simulink model "poly_festk2"  (Simulink 7.8)
settings: Solver=VariableStepDiscrete  StartTime=0.0  StopTime=100  RelTol=1e-3
undefined symbols (not defined in the file or in its folder): get
libraries: dspsigops x2, dspmlti4 x2, dspstat3 x1, dspsnks4 x1
settings Model: Creator=svenhoffmann  LastModifiedBy=josef  ExtModeAutoUpdateStatusClock=off
settings OptimizationCC: InitFltsAndDblsToZero=on
settings DebuggingCC: SaveWithParameterizedLinksMsg=none  SignalResolutionControl=TryResolveAllWithWarning  MultiTaskDSMMsg=warning  MultiTaskCondExecSysMsg=none  FcnCallInpInsideContextMsg=Use local settings  StrictBusMsg=None
settings RTWCC: IncludeERTFirstTime=on
settings GRTTargetCC: TargetFcnLib=ansi_tfl_tmw.mat

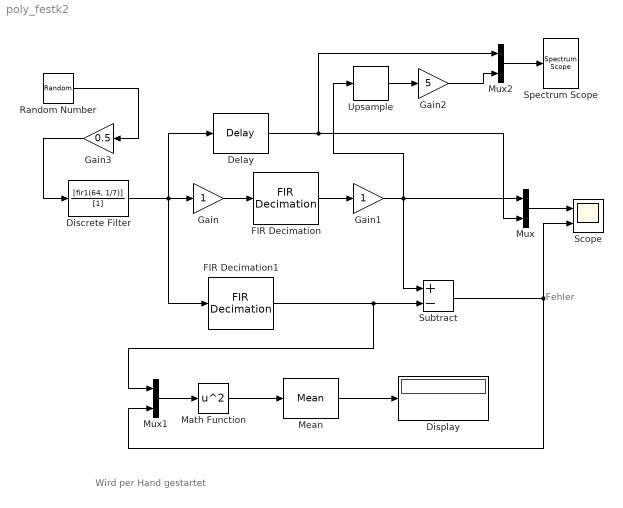
== system poly_festk2 ==
  note: Wird per Hand gestartet
  note: Fehler
  Delay : dspsigops/Delay  InputProcessing=Inherited (this choice will be removed - see release notes)  dly_unit=Samples  delay=64  ic_detail=off  dif_ic_for_ch=off  dif_ic_for_dly=off  ic=0  reset_popup=None
  Discrete Filter : DiscreteFilter  Numerator=[fir1(64, 1/7)]  Denominator=[1]
  Display : Display
  FIR Decimation : dspmlti4/FIR Decimation  h=fir1(128, 1/6)  D=5  filtStruct=Direct form  framing=Maintain input frame size  inputOffset=0  outputBufInitCond=0  InputProcessing=Inherited (this choice will be removed - see release notes)  firstCoeffMode=Binary point scaling  firstCoeffWordLength=16  firstCoeffFracLength=15  firstCoeffDataTypeStr=fixdt(1,16,15)  firstCoeffLastDataTypeStr=fixdt(1,16,15)  firstCoeffMin=[]  firstCoeffMax=[]  outputMin=[]  outputMax=[]  accumMode=Binary point scaling  accumWordLength=32  accumFracLength=30  accumDataTypeStr=fixdt(1,32,30)  accumLastDataTypeStr=fixdt(1,32,30)  prodOutputMode=Binary point scaling  prodOutputWordLength=32  prodOutputFracLength=30  prodOutputDataTypeStr=fixdt(1,32,30)  prodOutputLastDataTypeStr=fixdt(1,32,30)  roundingMode=Nearest  overflowMode=on  FilterSource=Specify via dialog  FilterObject=Hm_firdecim
  FIR Decimation1 : dspmlti4/FIR Decimation  h=fir1(128, 1/6)  D=5  filtStruct=Direct form  framing=Maintain input frame size  inputOffset=0  outputBufInitCond=0  InputProcessing=Inherited (this choice will be removed - see release notes)  firstCoeffMode=Binary point scaling  firstCoeffWordLength=16  firstCoeffFracLength=14  firstCoeffDataTypeStr=fixdt(1,16,14)  firstCoeffLastDataTypeStr=fixdt(1,16,14)  firstCoeffMin=[]  firstCoeffMax=[]  outputMode=Binary point scaling  outputWordLength=16  outputFracLength=14  outputDataTypeStr=fixdt(1,16,14)  outputLastDataTypeStr=fixdt(1,16,14)  outputMin=[]  outputMax=[]  accumDataTypeStr=Inherit: Same as product output  accumLastDataTypeStr=Inherit: Same as product output  prodOutputMode=Binary point scaling  prodOutputWordLength=32  prodOutputFracLength=28  prodOutputDataTypeStr=fixdt(1,32,28)  prodOutputLastDataTypeStr=fixdt(1,32,28)  roundingMode=Floor  overflowMode=off  FilterSource=Specify via dialog  FilterObject=Hm_firdecim
  Gain : Gain  OutDataTypeStr=fixdt(1,16,15)  RndMeth=Nearest
  Gain1 : Gain  OutDataTypeStr=Inherit: Inherit via back propagation  RndMeth=Nearest
  Gain2 : Gain  Gain=5
  Gain3 : Gain  Gain=0.5
  Math Function : Math  Operator=square  SaturateOnIntegerOverflow=on
  Mean : dspstat3/Mean  run=on  reset_popup=None  InputProcessing=Inherited (this choice will be removed - see release notes)  directionMode=Each column  dimension=1  treatSBRowAsCol=on  roiEnable=off  roiType=Rectangles  roiPortion=Entire ROI  roiOutput=Individual statistics for each ROI  roiFlag=off  outputDataTypeStr=Inherit: Same as accumulator  outputLastDataTypeStr=Inherit: Same as accumulator  outputMin=[]  outputMax=[]  roundingMode=Floor  overflowMode=off
  Mux : Mux  Inputs=2
  Mux1 : Mux  Inputs=2
  Mux2 : Mux  Inputs=2
  Random Number : RandomNumber  SampleTime=1/1000
  Scope : Scope  NumInputPorts=2
      settings: YMin=-0.8~-0.00015  YMax=0.9~0.00015
  Spectrum Scope : dspsnks4/Spectrum Scope  ScopeProperties=on  Domain=Frequency  HorizSpan=1  UseBuffer=on  BufferSize=256  Overlap=0  TreatMby1Signals=M channels  inpFftLenInherit=on  FFTlength=256  numAvg=10  DisplayProperties=off  AxisGrid=on  Memory=off  FrameNumber=on  AxisLegend=off  AxisZoom=off  OpenScopeAtSimStart=on  OpenScopeImmediately=off  FigPos=get(0,'defaultfigureposition')  AxisProperties=off  XUnits=Hertz  XRange=[0...Fs]  XDisplay=0  InheritXIncr=off  XIncr=1/1000  XLabel=Samples  XLimit=Auto  YUnits=dBW/Hertz  XMax=1  XMin=0  YLabel=Magnitude-squared, dB  LineProperties=off  wintypeSpecScope=Hann  RsSpecScope=50  betaSpecScope=5  winsampSpecScope=Periodic  XAxisParamsVer=6.8  isFrameUpgraded=on
      settings: YMin=-109.2182  YMax=-28.0292
  Subtract : Sum  Inputs=+-
  Upsample : dspsigops/Upsample  N=5  phase=0  InputProcessing=Inherited (this choice will be removed - see release notes)  RateOptions=Allow multirate processing  ic=0  mode=Unused parameter value
  wires:
  Discrete Filter/1 -> Gain/1, FIR Decimation1/1, Delay/1
  Gain/1 -> FIR Decimation/1
  FIR Decimation/1 -> Gain1/1
  Gain1/1 -> Subtract/1, Upsample/1, Mux/1
  Mux/1 -> Scope/1
  Delay/1 -> Mux/2, Mux2/1
  FIR Decimation1/1 -> Subtract/2, Mux1/1
  Subtract/1 -> Scope/2, Mux1/2
  Math Function/1 -> Mean/1
  Mean/1 -> Display/1
  Mux1/1 -> Math Function/1
  Mux2/1 -> Spectrum Scope/1
  Upsample/1 -> Gain2/1
  Gain2/1 -> Mux2/2
  Random Number/1 -> Gain3/1
  Gain3/1 -> Discrete Filter/1
